simulink model "model3"  (R2020a)
settings: Solver=VariableStepAuto  StartTime=0.0  StopTime=100  RelTol=1e-3
settings Model: Creator=11196  LastModifiedBy=11196

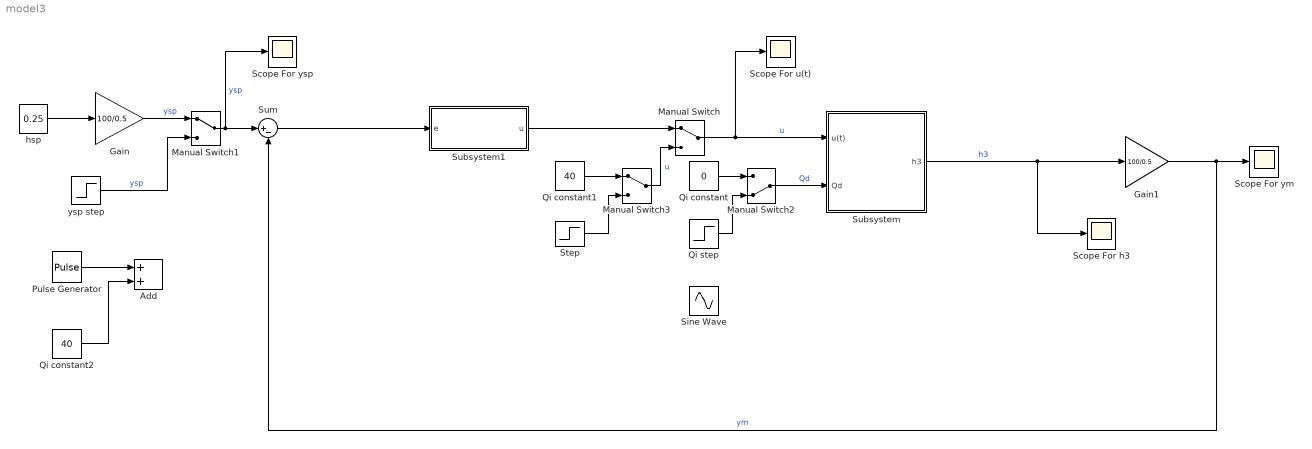
== system model3 ==
  Add : Sum
  Gain : Gain  Gain=100/0.5
  Gain1 : Gain  Gain=100/0.5
  Manual Switch : ManualSwitch
  Manual Switch1 : ManualSwitch
  Manual Switch2 : ManualSwitch  CurrentSetting=0
  Manual Switch3 : ManualSwitch
  Pulse Generator : DiscretePulseGenerator  PulseType=Time based  Amplitude=20  Period=5.5  PulseWidth=50
  Qi constant : Constant  Value=0
  Qi constant1 : Constant  Value=40
  Qi constant2 : Constant  Value=40
  Qi step : Step  Time=20  After=0.005  SampleTime=0
  Scope For h3 : Scope
  Scope For u(t) : Scope
  Scope For ym : Scope
  Scope For ysp : Scope
  Sine Wave : Sin  Amplitude=0.16  Frequency=0.5  SampleTime=0
  Step : Step  Time=20  Before=40  After=48  SampleTime=0
  Subsystem : Subsystem
  Subsystem1 : Subsystem
  Sum : Sum  Inputs=|+-
  hsp : Constant  Value=0.25
  ysp step : Step  Time=20  Before=50  After=59  SampleTime=0
  wires:
  Manual Switch2/1 -> Subsystem/2(Qd)  "Qd"
  Subsystem1/1(u) -> Manual Switch/1
  Gain1/1 -> Sum/2, Scope For ym/1  "ym"
  Step/1 -> Manual Switch3/2
  Manual Switch3/1 -> Manual Switch/2  "u"
  Gain/1 -> Manual Switch1/1  "ysp"
  Qi constant/1 -> Manual Switch2/1
  Manual Switch/1 -> Scope For u(t)/1, Subsystem/1(u(t))  "u"
  hsp/1 -> Gain/1
  Sum/1 -> Subsystem1/1(e)
  Manual Switch1/1 -> Scope For ysp/1, Sum/1  "ysp"
  Subsystem/1(h3) -> Scope For h3/1, Gain1/1  "h3"
  Qi constant1/1 -> Manual Switch3/1
  Qi step/1 -> Manual Switch2/2
  Pulse Generator/1 -> Add/1
  Qi constant2/1 -> Add/2
  ysp step/1 -> Manual Switch1/2  "ysp"

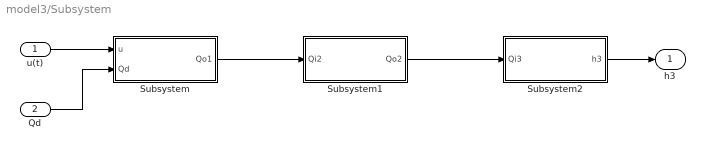
== system model3/Subsystem ==
  u(t) : Inport
  Qd : Inport  Port=2
  Subsystem : Subsystem
  Subsystem1 : Subsystem
  Subsystem2 : Subsystem
  h3 : Outport
  wires:
  Subsystem/1(Qo1) -> Subsystem1/1(Qi2)
  Subsystem1/1(Qo2) -> Subsystem2/1(Qi3)
  u(t)/1 -> Subsystem/1(u)
  Qd/1 -> Subsystem/2(Qd)
  Subsystem2/1(h3) -> h3/1

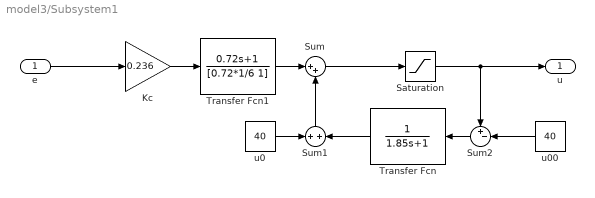
== system model3/Subsystem1 ==
  e : Inport
  Kc : Gain  Gain=0.236
  Saturation : Saturate  UpperLimit=100  LowerLimit=0
  Sum : Sum  Inputs=|++
  Sum1 : Sum  Inputs=+|+
  Sum2 : Sum  Inputs=+-|
  Transfer Fcn : TransferFcn  Denominator=[1.85 1]
  Transfer Fcn1 : TransferFcn  Numerator=[0.72 1]  Denominator=[0.72*1/6 1]
  u0 : Constant  Value=40
  u00 : Constant  Value=40
  u : Outport
  wires:
  e/1 -> Kc/1
  Sum/1 -> Saturation/1
  Saturation/1 -> Sum2/1, u/1
  u00/1 -> Sum2/2
  u0/1 -> Sum1/1
  Sum2/1 -> Transfer Fcn/1
  Transfer Fcn/1 -> Sum1/2
  Sum1/1 -> Sum/2
  Kc/1 -> Transfer Fcn1/1
  Transfer Fcn1/1 -> Sum/1

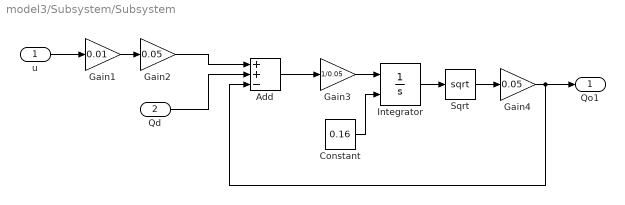
== system model3/Subsystem/Subsystem ==
  u : Inport
  Qd : Inport  Port=2
  Add : Sum  Inputs=++-
  Constant : Constant  Value=0.16
  Gain1 : Gain  Gain=0.01
  Gain2 : Gain  Gain=0.05
  Gain3 : Gain  Gain=1/0.05
  Gain4 : Gain  Gain=0.05
  Integrator : Integrator  InitialConditionSource=external  InitialCondition=3  LimitOutput=on  UpperSaturationLimit=0.5  LowerSaturationLimit=0
  Sqrt : Sqrt  SaturateOnIntegerOverflow=on
  Qo1 : Outport
  wires:
  u/1 -> Gain1/1
  Gain1/1 -> Gain2/1
  Gain2/1 -> Add/1
  Qd/1 -> Add/2
  Add/1 -> Gain3/1
  Gain3/1 -> Integrator/1
  Constant/1 -> Integrator/2
  Integrator/1 -> Sqrt/1
  Sqrt/1 -> Gain4/1
  Gain4/1 -> Add/3, Qo1/1

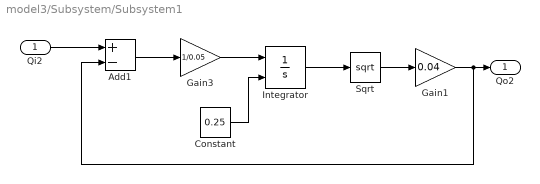
== system model3/Subsystem/Subsystem1 ==
  Qi2 : Inport
  Add1 : Sum  Inputs=+-
  Constant : Constant  Value=0.25
  Gain1 : Gain  Gain=0.04
  Gain3 : Gain  Gain=1/0.05
  Integrator : Integrator  InitialConditionSource=external  InitialCondition=3  LimitOutput=on  UpperSaturationLimit=0.5  LowerSaturationLimit=0
  Sqrt : Sqrt  SaturateOnIntegerOverflow=on
  Qo2 : Outport
  wires:
  Qi2/1 -> Add1/1
  Add1/1 -> Gain3/1
  Constant/1 -> Integrator/2
  Gain3/1 -> Integrator/1
  Integrator/1 -> Sqrt/1
  Sqrt/1 -> Gain1/1
  Gain1/1 -> Add1/2, Qo2/1

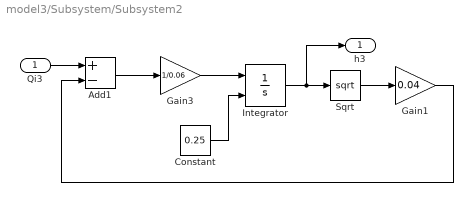
== system model3/Subsystem/Subsystem2 ==
  Qi3 : Inport
  Add1 : Sum  Inputs=+-
  Constant : Constant  Value=0.25
  Gain1 : Gain  Gain=0.04
  Gain3 : Gain  Gain=1/0.06
  Integrator : Integrator  InitialConditionSource=external  InitialCondition=3  LimitOutput=on  UpperSaturationLimit=0.5  LowerSaturationLimit=0
  Sqrt : Sqrt  SaturateOnIntegerOverflow=on
  h3 : Outport
  wires:
  Sqrt/1 -> Gain1/1
  Add1/1 -> Gain3/1
  Constant/1 -> Integrator/2
  Gain3/1 -> Integrator/1
  Integrator/1 -> h3/1, Sqrt/1
  Qi3/1 -> Add1/1
  Gain1/1 -> Add1/2
